simulink model "Heart_43N54P11VM_Waves"  (R2023b)
settings: Solver=ode1  StartTime=0.0  StopTime=30.0  FixedStep=0.5e-3  RelTol=1e-3
model workspace: external: MAT-File C:\Users\wai484\OneDrive - The University of Auckland\Documents\HeartModelPub\models_refine\N3Data_second_43N54P11VM.mat (data not in the file)
libraries: Libs_second x152
(part 1 of 3)
settings Model: SimulationMode=rapid-accelerator  Creator=wai484  LastModifiedBy=wai484
settings SolverCC: AlgebraicLoopSolver=TrustRegion
settings DataIOCC: SaveOutput=off  SignalLogging=off  DSMLogging=off  SaveTime=off  ReturnWorkspaceOutputs=off
settings DebuggingCC: UnconnectedInputMsg=warning  UnconnectedOutputMsg=warning  UnconnectedLineMsg=warning  ArithmeticOperatorsInVariantConditions=warning
settings ModelReferenceCC: EnableRefExpFcnMdlSchedulingChecks=on
settings SFSimCC: SimUseLocalCustomCode=off  CustomCodeUndefinedFunction=UseInterfaceOnly
settings RTWCC: RTWUseLocalCustomCode=off  BuildConfiguration=Faster Runs
settings CodeAppCC: StateflowObjectComments=on

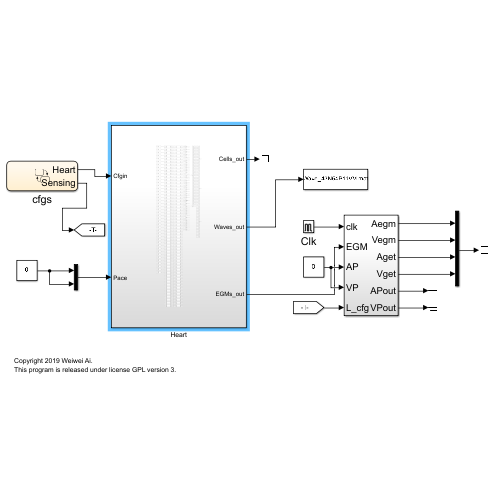
[thumbnail: Simulink's stored preview of the top-level diagram]
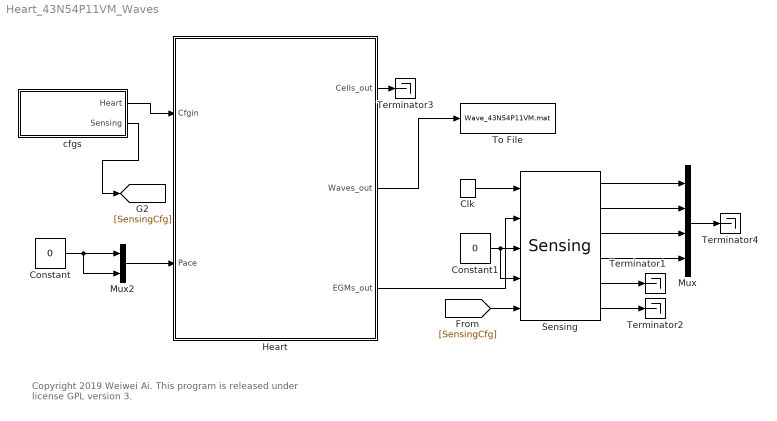
== system Heart_43N54P11VM_Waves ==
  note: Copyright 2019 Weiwei Ai.
      | This program is released under license GPL version 3.
  Clk : DiscretePulseGenerator  PulseType=Time based  Period=0.001  PulseWidth=50
  Constant : Constant  Value=0
  Constant1 : Constant  Value=0
  Heart : Subsystem
  Mux : Mux
  Mux2 : Mux  Inputs=2
  Sensing : Libs_second/Sensing  SystemSampleTime=-1  VariantActivationTime=update diagram  AllowFlexibleInterface=on  Latency=0  AutoFrameSizeCalculation=off
  Terminator{1..4} (4 alike) : Terminator
  To File : ToFile  Filename=Wave_43N54P11VM.mat  MatrixName=wave
  cfgs : Stateflow chart  TreatAsAtomicUnit=on
  wires:
  cfgs/1(Heart) -> Heart/1(Cfgin)
  Mux2/1 -> Heart/2(Pace)
  Constant/1 -> Mux2/2, Mux2/1
  Heart/2(Waves_out) -> To File/1
  Heart/3(EGMs_out) -> Sensing/2
  Sensing/5 -> Terminator1/1
  Constant1/1 -> Sensing/4, Sensing/3
  Clk/1 -> Sensing/1
  cfgs/2(Sensing) -> [SensingCfg]
  [SensingCfg] -> Sensing/5
  Sensing/6 -> Terminator2/1
  Sensing/1 -> Mux/1
  Sensing/2 -> Mux/2
  Sensing/3 -> Mux/3
  Sensing/4 -> Mux/4
  Heart/1(Cells_out) -> Terminator3/1
  Mux/1 -> Terminator4/1
